simulink model "pv_array2"  (R2015a)
settings: Solver=ode45  StartTime=0.0  StopTime=10  RelTol=1e-3
undefined symbols (not defined in the file or in its folder): sigbuilder_block
libraries: powerlib x24
(part 1 of 2)
settings Model: Creator=Limon  LastModifiedBy=Limon

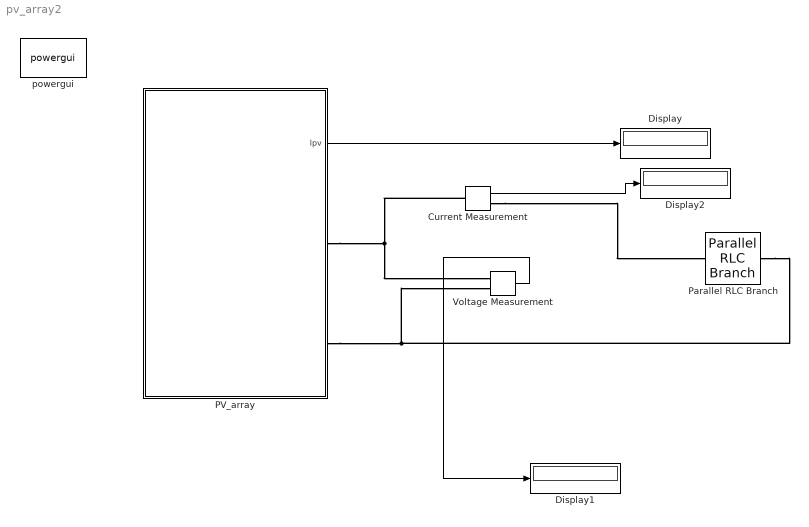
== system pv_array2 ==
  Current Measurement : powerlib/Measurements/Current Measurement  PhasorSimulation=off  OutputType=Complex  PSBequivalent=0
  Display : Display
  Display1 : Display
  Display2 : Display
  "PV_array " : Subsystem
  Parallel RLC Branch : powerlib/Elements/Parallel RLC Branch  LConnTagsString=a  RConnTagsString=__new0  BranchType=R  Resistance=1e3  Inductance=1e-3  SetiL0=off  InitialCurrent=0  Capacitance=1e-6  Setx0=off  InitialVoltage=0  Measurements=None
  Voltage Measurement : powerlib/Measurements/Voltage Measurement  PhasorSimulation=off  OutputType=Complex  PSBequivalent=0
  powergui : powerlib/powergui  Priority=1  SimulationMode=Discrete  SolverType=Tustin  SampleTime=.01  frequency=60  SPID=off  DisableSnubberDevices=off  DisableRonSwitches=off  DisableVfSwitches=off  SwTol=0  DisplayEquations=off  Interpol=off  methode=off  Ts=100  FunctionMessages=off  echomessages=off  HookPort=off  EnableUseOfTLC=off  x0status=blocks  frequencyindice=0  Pbase=100e6  ErrMax=0.0001  Iterations=50  UnitsV=kV  UnitsW=MW  buscounter=0  RestoreLinks=warning  ResistiveCurrentMeasurement=off  Frange=[0:2:500]  Ylog=off  Xlog=on  ShowGrid=off  save=off  variable=ZData  structure=MLFCDSTAT  ZoomFFT=off  StartTime=0.8  cycles=10  DisplayStyle=1  fundamental=50  FreqAxis=on  MaxFrequency=50000  frequencyindicesteady=1  RmsSteady=1  display=off
  wires:
  "PV_array "/1(Ipv) -> Display/1
  Voltage Measurement/1 -> Display1/1
  Current Measurement/1 -> Display2/1
  connections:
  "PV_array "/RConn1 -- Current Measurement/LConn1 -- Voltage Measurement/LConn1
  "PV_array "/RConn2 -- Parallel RLC Branch/RConn1 -- Voltage Measurement/LConn2
  Current Measurement/RConn1 -- Parallel RLC Branch/LConn1

== system pv_array2/PV_array  ==
  Irradiation : Subsystem
  PV module1 : Subsystem
  PV module10 : Subsystem
  PV module2 : Subsystem
  PV module3 : Subsystem
  PV module4 : Subsystem
  PV module5 : Subsystem
  PV module6 : Subsystem
  PV module7 : Subsystem
  PV module8 : Subsystem
  PV module9 : Subsystem
  + : PMIOPort  Port=1  Side=Right
  - : PMIOPort  Port=2  Side=Right
  Ipv : Outport
  wires:
  Irradiation/1(Irradiation) -> PV module1/1(Irradiation), PV module7/1(Irradiation), PV module10/1(Irradiation), PV module9/1(Irradiation), PV module5/1(Irradiation), PV module6/1(Irradiation), PV module8/1(Irradiation), PV module3/1(Irradiation), PV module4/1(Irradiation), PV module2/1(Irradiation)
  PV module9/1(Ipv) -> Ipv/1
  connections:
  PV module6/RConn1 -- PV module7/LConn1
  PV module9/RConn1 -- PV module10/LConn1
  PV module10/RConn1 -- PV module3/LConn1
  PV module5/RConn1 -- PV module6/LConn1
  PV module8/RConn1 -- -/RConn1
  PV module1/RConn1 -- PV module2/LConn1
  PV module9/LConn1 -- +/RConn1
  PV module4/LConn1 -- PV module2/RConn1
  PV module4/RConn1 -- PV module5/LConn1
  PV module1/LConn1 -- PV module3/RConn1
  PV module7/RConn1 -- PV module8/LConn1

== system pv_array2/PV_array /Irradiation ==
  Gain : Gain  Gain=1000
  Signal Builder : Subsystem  Tag=STV Subsys  LoadFcn=sigbuilder_block('load');  StartFcn=sigbuilder_block('start');  StopFcn=sigbuilder_block('stop');  ClipboardFcn=sigbuilder_block('clipboard');  mask(Sigbuilder block){}
      mask help: Simulink:masks:SigbuilderBlock_MD
      mask init:
      | if ~strcmp(get_param(bdroot(gcbh),'SimulationStatus'),'stopped') tuvar = sigbuilder_block('maskInit'); end
      settings: CopyFcn=sigbuilder_block('copy');  DeleteFcn=sigbuilder_block('delete');  ModelCloseFcn=sigbuilder_block('modelClose');  PreSaveFcn=sigbuilder_block('preSave');  PauseFcn=sigbuilder_block('pause');  ContinueFcn=sigbuilder_block('continue');  NameChangeFcn=sigbuilder_block('namechange');  OpenFcn=sigbuilder_block('open',[437.6 199.2 550.4 400 ]);  CloseFcn=sigbuilder_block('close');
      mask Display: plot(0, 0, 100, 100,[2, 2, 32, 32, 2], [68, 8, 8, 68, 68],[32, 2], [38, 38], [32, 19, 2],[53, 60, 44], [32, 17, 17, 2],[16, 16, 31, 31]);txt = getActiveGroup(gcbh);text(2, 100, txt,'verticalAlignment', 'top');
  Irradiation : Outport
  wires:
  Signal Builder/1(Signal 1) -> Gain/1
  Gain/1 -> Irradiation/1

== system pv_array2/PV_array /PV module1 ==
  Irradiation : Inport
  Display2 : Display
  PV module : Subsystem
  Temperature : Constant  Value=25
  VM1 : powerlib/Measurements/Voltage Measurement  PhasorSimulation=off  OutputType=Complex  PSBequivalent=0
  + : PMIOPort  Tag=PMCPort  Port=1  Side=Left
  - : PMIOPort  Tag=PMCPort  Port=2  Side=Right
  wires:
  Irradiation/1 -> PV module/2(Insol)
  Temperature/1 -> PV module/1(Temp)
  VM1/1 -> Display2/1
  connections:
  VM1/LConn1 -- +/RConn1 -- PV module/LConn1
  -/RConn1 -- VM1/LConn2 -- PV module/RConn1

== system pv_array2/PV_array /PV module10 ==
  Irradiation : Inport
  Display2 : Display
  PV module : Subsystem
  Temperature : Constant  Value=25
  VM1 : powerlib/Measurements/Voltage Measurement  PhasorSimulation=off  OutputType=Complex  PSBequivalent=0
  + : PMIOPort  Tag=PMCPort  Port=1  Side=Left
  - : PMIOPort  Tag=PMCPort  Port=2  Side=Right
  wires:
  Irradiation/1 -> PV module/2(Insol)
  Temperature/1 -> PV module/1(Temp)
  VM1/1 -> Display2/1
  connections:
  VM1/LConn1 -- +/RConn1 -- PV module/LConn1
  -/RConn1 -- VM1/LConn2 -- PV module/RConn1

== system pv_array2/PV_array /PV module2 ==
  Irradiation : Inport
  Display2 : Display
  PV module : Subsystem
  Temperature : Constant  Value=25
  VM1 : powerlib/Measurements/Voltage Measurement  PhasorSimulation=off  OutputType=Complex  PSBequivalent=0
  + : PMIOPort  Tag=PMCPort  Port=1  Side=Left
  - : PMIOPort  Tag=PMCPort  Port=2  Side=Right
  wires:
  Irradiation/1 -> PV module/2(Insol)
  Temperature/1 -> PV module/1(Temp)
  VM1/1 -> Display2/1
  connections:
  VM1/LConn1 -- +/RConn1 -- PV module/LConn1
  -/RConn1 -- VM1/LConn2 -- PV module/RConn1

== system pv_array2/PV_array /PV module3 ==
  Irradiation : Inport
  Display2 : Display
  PV module : Subsystem
  Temperature : Constant  Value=25
  VM1 : powerlib/Measurements/Voltage Measurement  PhasorSimulation=off  OutputType=Complex  PSBequivalent=0
  + : PMIOPort  Tag=PMCPort  Port=1  Side=Left
  - : PMIOPort  Tag=PMCPort  Port=2  Side=Right
  wires:
  Irradiation/1 -> PV module/2(Insol)
  Temperature/1 -> PV module/1(Temp)
  VM1/1 -> Display2/1
  connections:
  VM1/LConn1 -- +/RConn1 -- PV module/LConn1
  -/RConn1 -- VM1/LConn2 -- PV module/RConn1

== system pv_array2/PV_array /PV module4 ==
  Irradiation : Inport
  Display2 : Display
  PV module : Subsystem
  Temperature : Constant  Value=25
  VM1 : powerlib/Measurements/Voltage Measurement  PhasorSimulation=off  OutputType=Complex  PSBequivalent=0
  + : PMIOPort  Tag=PMCPort  Port=1  Side=Left
  - : PMIOPort  Tag=PMCPort  Port=2  Side=Right
  wires:
  Irradiation/1 -> PV module/2(Insol)
  Temperature/1 -> PV module/1(Temp)
  VM1/1 -> Display2/1
  connections:
  VM1/LConn1 -- +/RConn1 -- PV module/LConn1
  -/RConn1 -- VM1/LConn2 -- PV module/RConn1

== system pv_array2/PV_array /PV module5 ==
  Irradiation : Inport
  Display2 : Display
  PV module : Subsystem
  Temperature : Constant  Value=25
  VM1 : powerlib/Measurements/Voltage Measurement  PhasorSimulation=off  OutputType=Complex  PSBequivalent=0
  + : PMIOPort  Tag=PMCPort  Port=1  Side=Left
  - : PMIOPort  Tag=PMCPort  Port=2  Side=Right
  wires:
  Irradiation/1 -> PV module/2(Insol)
  Temperature/1 -> PV module/1(Temp)
  VM1/1 -> Display2/1
  connections:
  VM1/LConn1 -- +/RConn1 -- PV module/LConn1
  -/RConn1 -- VM1/LConn2 -- PV module/RConn1

== system pv_array2/PV_array /PV module6 ==
  Irradiation : Inport
  Display2 : Display
  PV module : Subsystem
  Temperature : Constant  Value=25
  VM1 : powerlib/Measurements/Voltage Measurement  PhasorSimulation=off  OutputType=Complex  PSBequivalent=0
  + : PMIOPort  Tag=PMCPort  Port=1  Side=Left
  - : PMIOPort  Tag=PMCPort  Port=2  Side=Right
  wires:
  Irradiation/1 -> PV module/2(Insol)
  Temperature/1 -> PV module/1(Temp)
  VM1/1 -> Display2/1
  connections:
  VM1/LConn1 -- +/RConn1 -- PV module/LConn1
  -/RConn1 -- VM1/LConn2 -- PV module/RConn1

== system pv_array2/PV_array /PV module7 ==
  Irradiation : Inport
  Display2 : Display
  PV module : Subsystem
  Temperature : Constant  Value=25
  VM1 : powerlib/Measurements/Voltage Measurement  PhasorSimulation=off  OutputType=Complex  PSBequivalent=0
  + : PMIOPort  Tag=PMCPort  Port=1  Side=Left
  - : PMIOPort  Tag=PMCPort  Port=2  Side=Right
  wires:
  Irradiation/1 -> PV module/2(Insol)
  Temperature/1 -> PV module/1(Temp)
  VM1/1 -> Display2/1
  connections:
  VM1/LConn1 -- +/RConn1 -- PV module/LConn1
  -/RConn1 -- VM1/LConn2 -- PV module/RConn1

== system pv_array2/PV_array /PV module8 ==
  Irradiation : Inport
  Display2 : Display
  PV module : Subsystem
  Temperature : Constant  Value=25
  VM1 : powerlib/Measurements/Voltage Measurement  PhasorSimulation=off  OutputType=Complex  PSBequivalent=0
  + : PMIOPort  Tag=PMCPort  Port=1  Side=Left
  - : PMIOPort  Tag=PMCPort  Port=2  Side=Right
  wires:
  Irradiation/1 -> PV module/2(Insol)
  Temperature/1 -> PV module/1(Temp)
  VM1/1 -> Display2/1
  connections:
  VM1/LConn1 -- +/RConn1 -- PV module/LConn1
  -/RConn1 -- VM1/LConn2 -- PV module/RConn1

== system pv_array2/PV_array /PV module9 ==
  Irradiation : Inport
  Display2 : Display
  PV module : Subsystem
  Temperature : Constant  Value=25
  VM1 : powerlib/Measurements/Voltage Measurement  PhasorSimulation=off  OutputType=Complex  PSBequivalent=0
  + : PMIOPort  Tag=PMCPort  Port=1  Side=Left
  - : PMIOPort  Tag=PMCPort  Port=2  Side=Right
  Ipv : Outport
  wires:
  Irradiation/1 -> PV module/2(Insol)
  Temperature/1 -> PV module/1(Temp)
  VM1/1 -> Display2/1
  PV module/1(Ipv) -> Ipv/1
  connections:
  VM1/LConn1 -- +/RConn1 -- PV module/LConn1
  -/RConn1 -- VM1/LConn2 -- PV module/RConn1

== system pv_array2/PV_array /Irradiation/Signal Builder ==
  Demux : Demux  Tag=STV Demux  Outputs=1
  FromWs : FromWorkspace  Tag=STV FromWs  VariableName=tuvar  SampleTime=0
      SigBuilderData=|
      | common.afterFinalStr = 'Extrapolate'
      | common.sampleTime = 0
      | dataSet.timeRange = [0 30]
      | dataSet.name = 'Group 1'
      | sbobj.Groups.Name = 'Group 1'
      | sbobj.Groups.Signals.Name = 'Signal 1'
      | sbobj.Groups.Signals.XData = [0 10 10 20 20 30]
      | sbobj.Groups.Signals.YData = [0.2 0.2 0.6 0.6 1 0.995]
      | sbobj.Groups.TimeRange = [0 30]
  Signal 1 : Outport  Tag=STV Outport
  wires:
  Demux/1 -> Signal 1/1
  FromWs/1 -> Demux/1

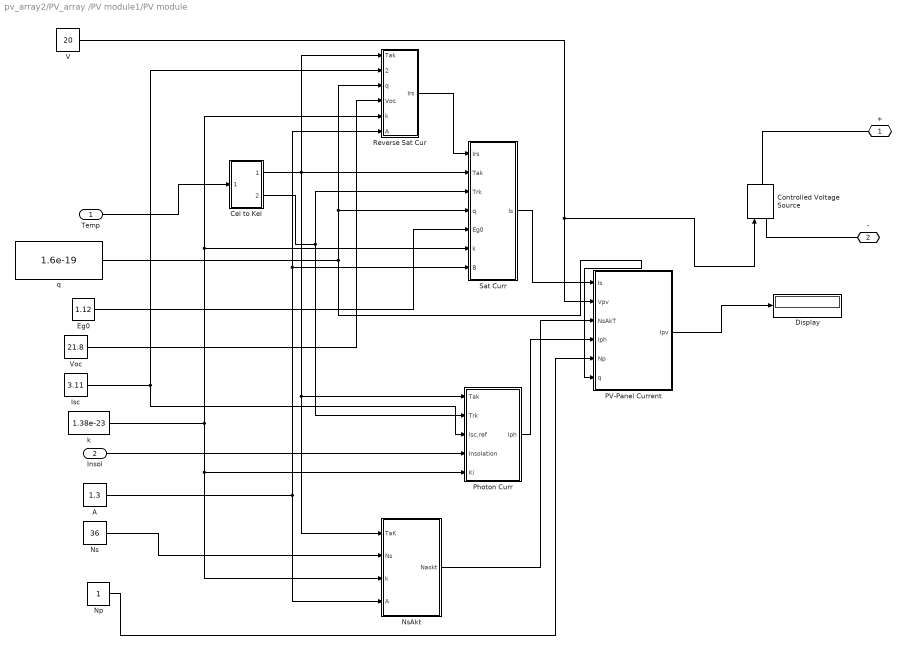
== system pv_array2/PV_array /PV module1/PV module ==
  Temp : Inport
  Insol : Inport  Port=2
  A : Constant  Value=1.3
  Cel to Kel : Subsystem
  Controlled Voltage Source : powerlib/Electrical Sources/Controlled Voltage Source  Initialize=on  Source_Type=AC  Amplitude=0  Phase=0  Frequency=0  Measurements=None
  Display : Display
  Eg0 : Constant  Value=1.12
  Isc : Constant  Value=3.11
  Np : Constant
  Ns : Constant  Value=36
  NsAkt : Subsystem
  PV-Panel Current : Subsystem
  "Photon Curr " : Subsystem
  "Reverse Sat Cur " : Subsystem
  Sat Curr : Subsystem
  V : Constant  Value=20
  Voc : Constant  Value=21.8
  k : Constant  Value=1.38e-23
  q : Constant  Value=1.6e-19
  + : PMIOPort  Port=1  Side=Left
  - : PMIOPort  Port=2  Side=Right
  wires:
  "Photon Curr "/1("Iph ") -> PV-Panel Current/4("Iph ")
  NsAkt/1(Naskt) -> PV-Panel Current/3(NsAkT)
  "Reverse Sat Cur "/1(Irs) -> Sat Curr/1(Irs)
  Cel to Kel/1("Tak ") -> "Photon Curr "/1("Tak "), NsAkt/1(TaK), "Reverse Sat Cur "/1("Tak "), Sat Curr/2(Tak)
  Sat Curr/1(Is) -> PV-Panel Current/1(Is)
  Temp/1 -> Cel to Kel/1("Top ")
  V/1 -> Controlled Voltage Source/1, PV-Panel Current/2("Vpv ")
  Ns/1 -> NsAkt/2(Ns)
  Cel to Kel/2("Trk ") -> "Photon Curr "/2(Trk), Sat Curr/3(Trk)
  Isc/1 -> "Reverse Sat Cur "/2("Isc ref "), "Photon Curr "/3(Isc,ref)
  q/1 -> Sat Curr/4(q), "Reverse Sat Cur "/3(q), PV-Panel Current/6(q)
  Voc/1 -> "Reverse Sat Cur "/4(Voc)
  k/1 -> Sat Curr/6(k), "Reverse Sat Cur "/5(k), NsAkt/3(k), "Photon Curr "/5(Ki)
  A/1 -> Sat Curr/7(B), "Reverse Sat Cur "/6("A "), NsAkt/4(A)
  Insol/1 -> "Photon Curr "/4("Insolation ")
  Np/1 -> PV-Panel Current/5(Np)
  Eg0/1 -> Sat Curr/5(Eg0)
  PV-Panel Current/1(Ipv) -> Display/1
  connections:
  +/RConn1 -- Controlled Voltage Source/RConn1
  -/RConn1 -- Controlled Voltage Source/LConn1

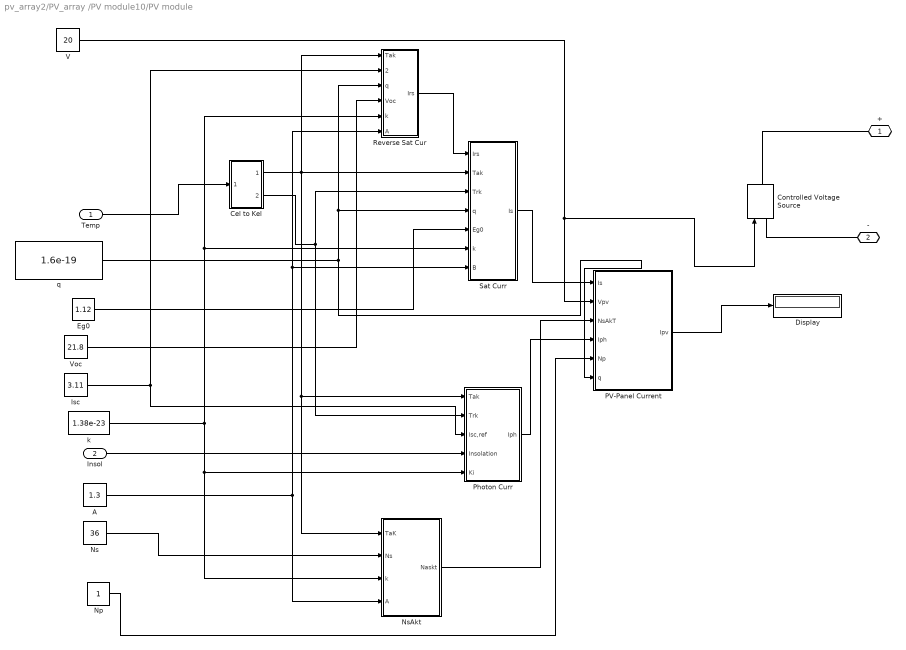
== system pv_array2/PV_array /PV module10/PV module ==
  Temp : Inport
  Insol : Inport  Port=2
  A : Constant  Value=1.3
  Cel to Kel : Subsystem
  Controlled Voltage Source : powerlib/Electrical Sources/Controlled Voltage Source  Initialize=on  Source_Type=AC  Amplitude=0  Phase=0  Frequency=0  Measurements=None
  Display : Display
  Eg0 : Constant  Value=1.12
  Isc : Constant  Value=3.11
  Np : Constant
  Ns : Constant  Value=36
  NsAkt : Subsystem
  PV-Panel Current : Subsystem
  "Photon Curr " : Subsystem
  "Reverse Sat Cur " : Subsystem
  Sat Curr : Subsystem
  V : Constant  Value=20
  Voc : Constant  Value=21.8
  k : Constant  Value=1.38e-23
  q : Constant  Value=1.6e-19
  + : PMIOPort  Port=1  Side=Left
  - : PMIOPort  Port=2  Side=Right
  wires:
  "Photon Curr "/1("Iph ") -> PV-Panel Current/4("Iph ")
  NsAkt/1(Naskt) -> PV-Panel Current/3(NsAkT)
  "Reverse Sat Cur "/1(Irs) -> Sat Curr/1(Irs)
  Cel to Kel/1("Tak ") -> "Photon Curr "/1("Tak "), NsAkt/1(TaK), "Reverse Sat Cur "/1("Tak "), Sat Curr/2(Tak)
  Sat Curr/1(Is) -> PV-Panel Current/1(Is)
  Temp/1 -> Cel to Kel/1("Top ")
  V/1 -> Controlled Voltage Source/1, PV-Panel Current/2("Vpv ")
  Ns/1 -> NsAkt/2(Ns)
  Cel to Kel/2("Trk ") -> "Photon Curr "/2(Trk), Sat Curr/3(Trk)
  Isc/1 -> "Reverse Sat Cur "/2("Isc ref "), "Photon Curr "/3(Isc,ref)
  q/1 -> Sat Curr/4(q), "Reverse Sat Cur "/3(q), PV-Panel Current/6(q)
  Voc/1 -> "Reverse Sat Cur "/4(Voc)
  k/1 -> Sat Curr/6(k), "Reverse Sat Cur "/5(k), NsAkt/3(k), "Photon Curr "/5(Ki)
  A/1 -> Sat Curr/7(B), "Reverse Sat Cur "/6("A "), NsAkt/4(A)
  Insol/1 -> "Photon Curr "/4("Insolation ")
  Np/1 -> PV-Panel Current/5(Np)
  Eg0/1 -> Sat Curr/5(Eg0)
  PV-Panel Current/1(Ipv) -> Display/1
  connections:
  +/RConn1 -- Controlled Voltage Source/RConn1
  -/RConn1 -- Controlled Voltage Source/LConn1

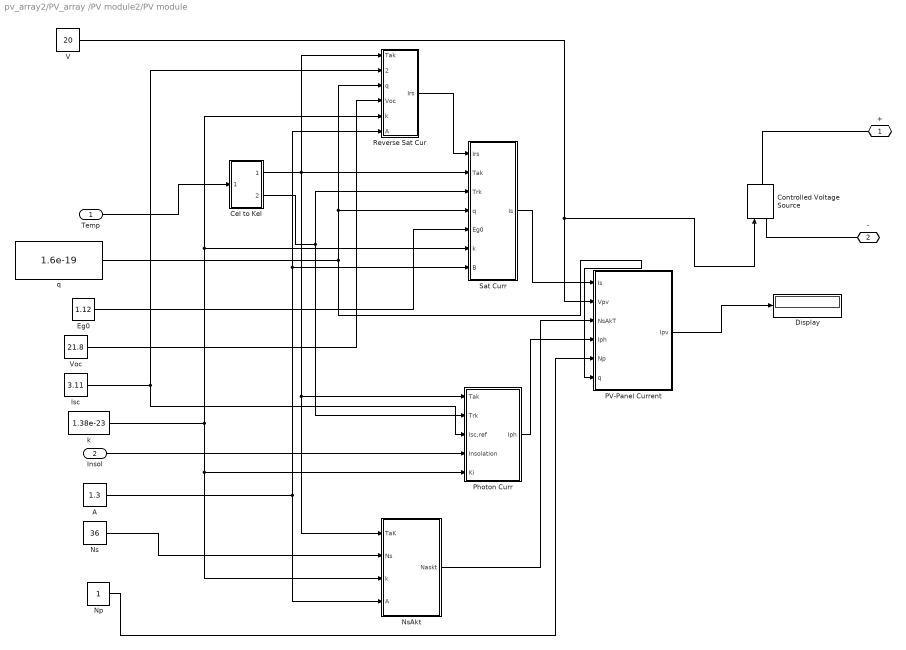
== system pv_array2/PV_array /PV module2/PV module ==
  Temp : Inport
  Insol : Inport  Port=2
  A : Constant  Value=1.3
  Cel to Kel : Subsystem
  Controlled Voltage Source : powerlib/Electrical Sources/Controlled Voltage Source  Initialize=on  Source_Type=AC  Amplitude=0  Phase=0  Frequency=0  Measurements=None
  Display : Display
  Eg0 : Constant  Value=1.12
  Isc : Constant  Value=3.11
  Np : Constant
  Ns : Constant  Value=36
  NsAkt : Subsystem
  PV-Panel Current : Subsystem
  "Photon Curr " : Subsystem
  "Reverse Sat Cur " : Subsystem
  Sat Curr : Subsystem
  V : Constant  Value=20
  Voc : Constant  Value=21.8
  k : Constant  Value=1.38e-23
  q : Constant  Value=1.6e-19
  + : PMIOPort  Port=1  Side=Left
  - : PMIOPort  Port=2  Side=Right
  wires:
  "Photon Curr "/1("Iph ") -> PV-Panel Current/4("Iph ")
  NsAkt/1(Naskt) -> PV-Panel Current/3(NsAkT)
  "Reverse Sat Cur "/1(Irs) -> Sat Curr/1(Irs)
  Cel to Kel/1("Tak ") -> "Photon Curr "/1("Tak "), NsAkt/1(TaK), "Reverse Sat Cur "/1("Tak "), Sat Curr/2(Tak)
  Sat Curr/1(Is) -> PV-Panel Current/1(Is)
  Temp/1 -> Cel to Kel/1("Top ")
  V/1 -> Controlled Voltage Source/1, PV-Panel Current/2("Vpv ")
  Ns/1 -> NsAkt/2(Ns)
  Cel to Kel/2("Trk ") -> "Photon Curr "/2(Trk), Sat Curr/3(Trk)
  Isc/1 -> "Reverse Sat Cur "/2("Isc ref "), "Photon Curr "/3(Isc,ref)
  q/1 -> Sat Curr/4(q), "Reverse Sat Cur "/3(q), PV-Panel Current/6(q)
  Voc/1 -> "Reverse Sat Cur "/4(Voc)
  k/1 -> Sat Curr/6(k), "Reverse Sat Cur "/5(k), NsAkt/3(k), "Photon Curr "/5(Ki)
  A/1 -> Sat Curr/7(B), "Reverse Sat Cur "/6("A "), NsAkt/4(A)
  Insol/1 -> "Photon Curr "/4("Insolation ")
  Np/1 -> PV-Panel Current/5(Np)
  Eg0/1 -> Sat Curr/5(Eg0)
  PV-Panel Current/1(Ipv) -> Display/1
  connections:
  +/RConn1 -- Controlled Voltage Source/RConn1
  -/RConn1 -- Controlled Voltage Source/LConn1

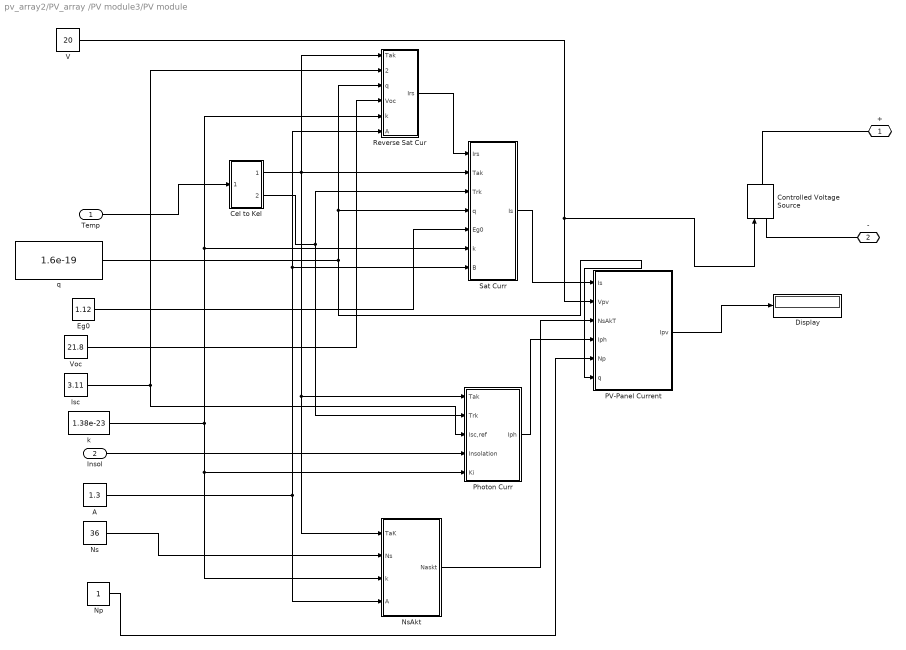
== system pv_array2/PV_array /PV module3/PV module ==
  Temp : Inport
  Insol : Inport  Port=2
  A : Constant  Value=1.3
  Cel to Kel : Subsystem
  Controlled Voltage Source : powerlib/Electrical Sources/Controlled Voltage Source  Initialize=on  Source_Type=AC  Amplitude=0  Phase=0  Frequency=0  Measurements=None
  Display : Display
  Eg0 : Constant  Value=1.12
  Isc : Constant  Value=3.11
  Np : Constant
  Ns : Constant  Value=36
  NsAkt : Subsystem
  PV-Panel Current : Subsystem
  "Photon Curr " : Subsystem
  "Reverse Sat Cur " : Subsystem
  Sat Curr : Subsystem
  V : Constant  Value=20
  Voc : Constant  Value=21.8
  k : Constant  Value=1.38e-23
  q : Constant  Value=1.6e-19
  + : PMIOPort  Port=1  Side=Left
  - : PMIOPort  Port=2  Side=Right
  wires:
  "Photon Curr "/1("Iph ") -> PV-Panel Current/4("Iph ")
  NsAkt/1(Naskt) -> PV-Panel Current/3(NsAkT)
  "Reverse Sat Cur "/1(Irs) -> Sat Curr/1(Irs)
  Cel to Kel/1("Tak ") -> "Photon Curr "/1("Tak "), NsAkt/1(TaK), "Reverse Sat Cur "/1("Tak "), Sat Curr/2(Tak)
  Sat Curr/1(Is) -> PV-Panel Current/1(Is)
  Temp/1 -> Cel to Kel/1("Top ")
  V/1 -> Controlled Voltage Source/1, PV-Panel Current/2("Vpv ")
  Ns/1 -> NsAkt/2(Ns)
  Cel to Kel/2("Trk ") -> "Photon Curr "/2(Trk), Sat Curr/3(Trk)
  Isc/1 -> "Reverse Sat Cur "/2("Isc ref "), "Photon Curr "/3(Isc,ref)
  q/1 -> Sat Curr/4(q), "Reverse Sat Cur "/3(q), PV-Panel Current/6(q)
  Voc/1 -> "Reverse Sat Cur "/4(Voc)
  k/1 -> Sat Curr/6(k), "Reverse Sat Cur "/5(k), NsAkt/3(k), "Photon Curr "/5(Ki)
  A/1 -> Sat Curr/7(B), "Reverse Sat Cur "/6("A "), NsAkt/4(A)
  Insol/1 -> "Photon Curr "/4("Insolation ")
  Np/1 -> PV-Panel Current/5(Np)
  Eg0/1 -> Sat Curr/5(Eg0)
  PV-Panel Current/1(Ipv) -> Display/1
  connections:
  +/RConn1 -- Controlled Voltage Source/RConn1
  -/RConn1 -- Controlled Voltage Source/LConn1

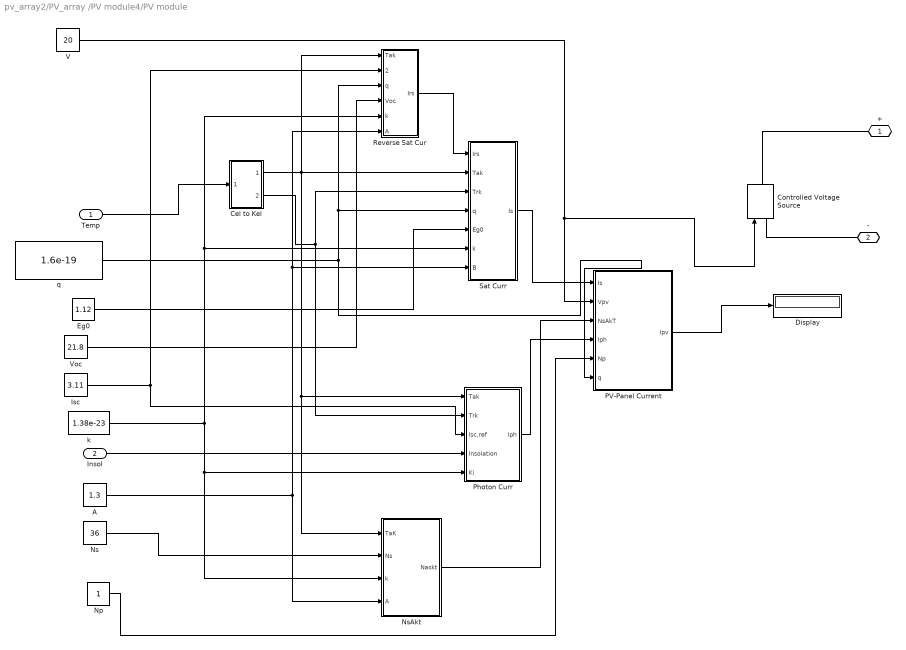
== system pv_array2/PV_array /PV module4/PV module ==
  Temp : Inport
  Insol : Inport  Port=2
  A : Constant  Value=1.3
  Cel to Kel : Subsystem
  Controlled Voltage Source : powerlib/Electrical Sources/Controlled Voltage Source  Initialize=on  Source_Type=AC  Amplitude=0  Phase=0  Frequency=0  Measurements=None
  Display : Display
  Eg0 : Constant  Value=1.12
  Isc : Constant  Value=3.11
  Np : Constant
  Ns : Constant  Value=36
  NsAkt : Subsystem
  PV-Panel Current : Subsystem
  "Photon Curr " : Subsystem
  "Reverse Sat Cur " : Subsystem
  Sat Curr : Subsystem
  V : Constant  Value=20
  Voc : Constant  Value=21.8
  k : Constant  Value=1.38e-23
  q : Constant  Value=1.6e-19
  + : PMIOPort  Port=1  Side=Left
  - : PMIOPort  Port=2  Side=Right
  wires:
  "Photon Curr "/1("Iph ") -> PV-Panel Current/4("Iph ")
  NsAkt/1(Naskt) -> PV-Panel Current/3(NsAkT)
  "Reverse Sat Cur "/1(Irs) -> Sat Curr/1(Irs)
  Cel to Kel/1("Tak ") -> "Photon Curr "/1("Tak "), NsAkt/1(TaK), "Reverse Sat Cur "/1("Tak "), Sat Curr/2(Tak)
  Sat Curr/1(Is) -> PV-Panel Current/1(Is)
  Temp/1 -> Cel to Kel/1("Top ")
  V/1 -> Controlled Voltage Source/1, PV-Panel Current/2("Vpv ")
  Ns/1 -> NsAkt/2(Ns)
  Cel to Kel/2("Trk ") -> "Photon Curr "/2(Trk), Sat Curr/3(Trk)
  Isc/1 -> "Reverse Sat Cur "/2("Isc ref "), "Photon Curr "/3(Isc,ref)
  q/1 -> Sat Curr/4(q), "Reverse Sat Cur "/3(q), PV-Panel Current/6(q)
  Voc/1 -> "Reverse Sat Cur "/4(Voc)
  k/1 -> Sat Curr/6(k), "Reverse Sat Cur "/5(k), NsAkt/3(k), "Photon Curr "/5(Ki)
  A/1 -> Sat Curr/7(B), "Reverse Sat Cur "/6("A "), NsAkt/4(A)
  Insol/1 -> "Photon Curr "/4("Insolation ")
  Np/1 -> PV-Panel Current/5(Np)
  Eg0/1 -> Sat Curr/5(Eg0)
  PV-Panel Current/1(Ipv) -> Display/1
  connections:
  +/RConn1 -- Controlled Voltage Source/RConn1
  -/RConn1 -- Controlled Voltage Source/LConn1

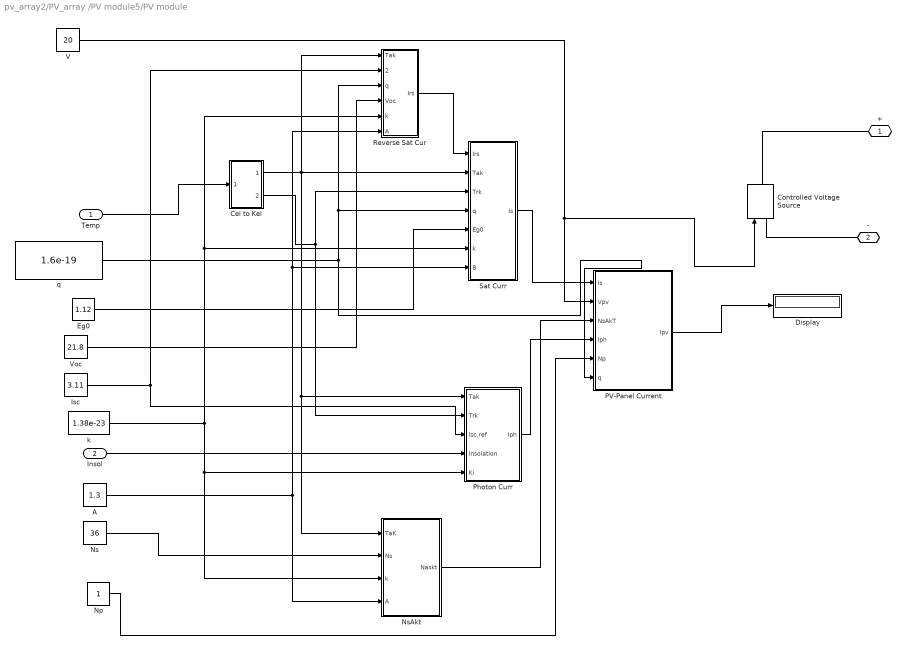
== system pv_array2/PV_array /PV module5/PV module ==
  Temp : Inport
  Insol : Inport  Port=2
  A : Constant  Value=1.3
  Cel to Kel : Subsystem
  Controlled Voltage Source : powerlib/Electrical Sources/Controlled Voltage Source  Initialize=on  Source_Type=AC  Amplitude=0  Phase=0  Frequency=0  Measurements=None
  Display : Display
  Eg0 : Constant  Value=1.12
  Isc : Constant  Value=3.11
  Np : Constant
  Ns : Constant  Value=36
  NsAkt : Subsystem
  PV-Panel Current : Subsystem
  "Photon Curr " : Subsystem
  "Reverse Sat Cur " : Subsystem
  Sat Curr : Subsystem
  V : Constant  Value=20
  Voc : Constant  Value=21.8
  k : Constant  Value=1.38e-23
  q : Constant  Value=1.6e-19
  + : PMIOPort  Port=1  Side=Left
  - : PMIOPort  Port=2  Side=Right
  wires:
  "Photon Curr "/1("Iph ") -> PV-Panel Current/4("Iph ")
  NsAkt/1(Naskt) -> PV-Panel Current/3(NsAkT)
  "Reverse Sat Cur "/1(Irs) -> Sat Curr/1(Irs)
  Cel to Kel/1("Tak ") -> "Photon Curr "/1("Tak "), NsAkt/1(TaK), "Reverse Sat Cur "/1("Tak "), Sat Curr/2(Tak)
  Sat Curr/1(Is) -> PV-Panel Current/1(Is)
  Temp/1 -> Cel to Kel/1("Top ")
  V/1 -> Controlled Voltage Source/1, PV-Panel Current/2("Vpv ")
  Ns/1 -> NsAkt/2(Ns)
  Cel to Kel/2("Trk ") -> "Photon Curr "/2(Trk), Sat Curr/3(Trk)
  Isc/1 -> "Reverse Sat Cur "/2("Isc ref "), "Photon Curr "/3(Isc,ref)
  q/1 -> Sat Curr/4(q), "Reverse Sat Cur "/3(q), PV-Panel Current/6(q)
  Voc/1 -> "Reverse Sat Cur "/4(Voc)
  k/1 -> Sat Curr/6(k), "Reverse Sat Cur "/5(k), NsAkt/3(k), "Photon Curr "/5(Ki)
  A/1 -> Sat Curr/7(B), "Reverse Sat Cur "/6("A "), NsAkt/4(A)
  Insol/1 -> "Photon Curr "/4("Insolation ")
  Np/1 -> PV-Panel Current/5(Np)
  Eg0/1 -> Sat Curr/5(Eg0)
  PV-Panel Current/1(Ipv) -> Display/1
  connections:
  +/RConn1 -- Controlled Voltage Source/RConn1
  -/RConn1 -- Controlled Voltage Source/LConn1

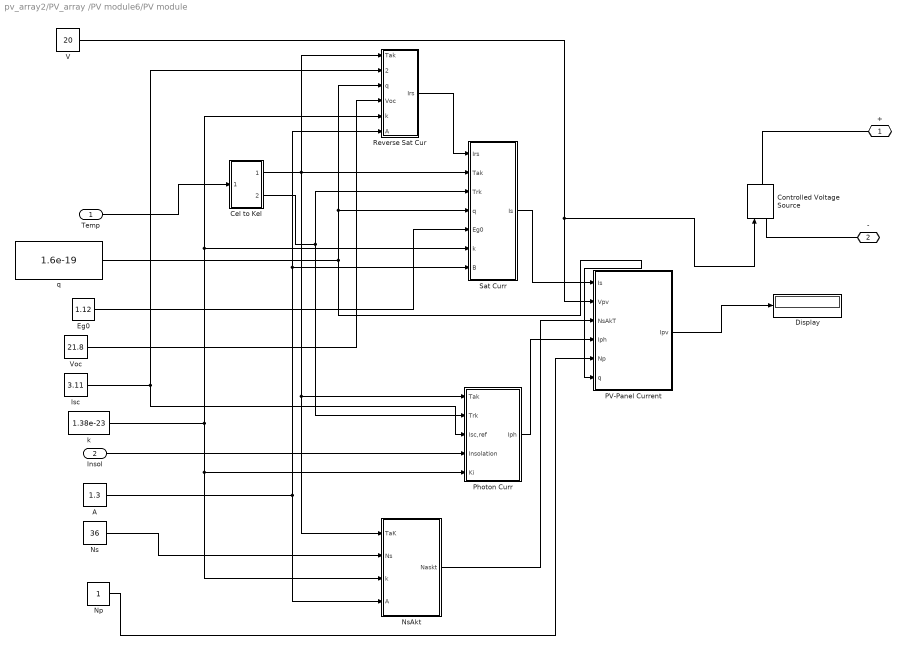
== system pv_array2/PV_array /PV module6/PV module ==
  Temp : Inport
  Insol : Inport  Port=2
  A : Constant  Value=1.3
  Cel to Kel : Subsystem
  Controlled Voltage Source : powerlib/Electrical Sources/Controlled Voltage Source  Initialize=on  Source_Type=AC  Amplitude=0  Phase=0  Frequency=0  Measurements=None
  Display : Display
  Eg0 : Constant  Value=1.12
  Isc : Constant  Value=3.11
  Np : Constant
  Ns : Constant  Value=36
  NsAkt : Subsystem
  PV-Panel Current : Subsystem
  "Photon Curr " : Subsystem
  "Reverse Sat Cur " : Subsystem
  Sat Curr : Subsystem
  V : Constant  Value=20
  Voc : Constant  Value=21.8
  k : Constant  Value=1.38e-23
  q : Constant  Value=1.6e-19
  + : PMIOPort  Port=1  Side=Left
  - : PMIOPort  Port=2  Side=Right
  wires:
  "Photon Curr "/1("Iph ") -> PV-Panel Current/4("Iph ")
  NsAkt/1(Naskt) -> PV-Panel Current/3(NsAkT)
  "Reverse Sat Cur "/1(Irs) -> Sat Curr/1(Irs)
  Cel to Kel/1("Tak ") -> "Photon Curr "/1("Tak "), NsAkt/1(TaK), "Reverse Sat Cur "/1("Tak "), Sat Curr/2(Tak)
  Sat Curr/1(Is) -> PV-Panel Current/1(Is)
  Temp/1 -> Cel to Kel/1("Top ")
  V/1 -> Controlled Voltage Source/1, PV-Panel Current/2("Vpv ")
  Ns/1 -> NsAkt/2(Ns)
  Cel to Kel/2("Trk ") -> "Photon Curr "/2(Trk), Sat Curr/3(Trk)
  Isc/1 -> "Reverse Sat Cur "/2("Isc ref "), "Photon Curr "/3(Isc,ref)
  q/1 -> Sat Curr/4(q), "Reverse Sat Cur "/3(q), PV-Panel Current/6(q)
  Voc/1 -> "Reverse Sat Cur "/4(Voc)
  k/1 -> Sat Curr/6(k), "Reverse Sat Cur "/5(k), NsAkt/3(k), "Photon Curr "/5(Ki)
  A/1 -> Sat Curr/7(B), "Reverse Sat Cur "/6("A "), NsAkt/4(A)
  Insol/1 -> "Photon Curr "/4("Insolation ")
  Np/1 -> PV-Panel Current/5(Np)
  Eg0/1 -> Sat Curr/5(Eg0)
  PV-Panel Current/1(Ipv) -> Display/1
  connections:
  +/RConn1 -- Controlled Voltage Source/RConn1
  -/RConn1 -- Controlled Voltage Source/LConn1

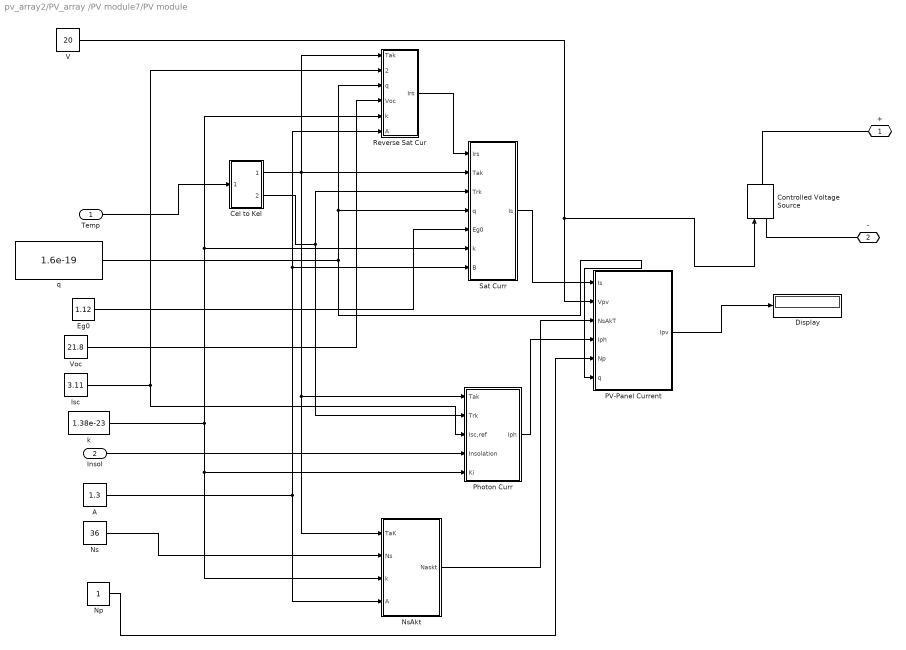
== system pv_array2/PV_array /PV module7/PV module ==
  Temp : Inport
  Insol : Inport  Port=2
  A : Constant  Value=1.3
  Cel to Kel : Subsystem
  Controlled Voltage Source : powerlib/Electrical Sources/Controlled Voltage Source  Initialize=on  Source_Type=AC  Amplitude=0  Phase=0  Frequency=0  Measurements=None
  Display : Display
  Eg0 : Constant  Value=1.12
  Isc : Constant  Value=3.11
  Np : Constant
  Ns : Constant  Value=36
  NsAkt : Subsystem
  PV-Panel Current : Subsystem
  "Photon Curr " : Subsystem
  "Reverse Sat Cur " : Subsystem
  Sat Curr : Subsystem
  V : Constant  Value=20
  Voc : Constant  Value=21.8
  k : Constant  Value=1.38e-23
  q : Constant  Value=1.6e-19
  + : PMIOPort  Port=1  Side=Left
  - : PMIOPort  Port=2  Side=Right
  wires:
  "Photon Curr "/1("Iph ") -> PV-Panel Current/4("Iph ")
  NsAkt/1(Naskt) -> PV-Panel Current/3(NsAkT)
  "Reverse Sat Cur "/1(Irs) -> Sat Curr/1(Irs)
  Cel to Kel/1("Tak ") -> "Photon Curr "/1("Tak "), NsAkt/1(TaK), "Reverse Sat Cur "/1("Tak "), Sat Curr/2(Tak)
  Sat Curr/1(Is) -> PV-Panel Current/1(Is)
  Temp/1 -> Cel to Kel/1("Top ")
  V/1 -> Controlled Voltage Source/1, PV-Panel Current/2("Vpv ")
  Ns/1 -> NsAkt/2(Ns)
  Cel to Kel/2("Trk ") -> "Photon Curr "/2(Trk), Sat Curr/3(Trk)
  Isc/1 -> "Reverse Sat Cur "/2("Isc ref "), "Photon Curr "/3(Isc,ref)
  q/1 -> Sat Curr/4(q), "Reverse Sat Cur "/3(q), PV-Panel Current/6(q)
  Voc/1 -> "Reverse Sat Cur "/4(Voc)
  k/1 -> Sat Curr/6(k), "Reverse Sat Cur "/5(k), NsAkt/3(k), "Photon Curr "/5(Ki)
  A/1 -> Sat Curr/7(B), "Reverse Sat Cur "/6("A "), NsAkt/4(A)
  Insol/1 -> "Photon Curr "/4("Insolation ")
  Np/1 -> PV-Panel Current/5(Np)
  Eg0/1 -> Sat Curr/5(Eg0)
  PV-Panel Current/1(Ipv) -> Display/1
  connections:
  +/RConn1 -- Controlled Voltage Source/RConn1
  -/RConn1 -- Controlled Voltage Source/LConn1

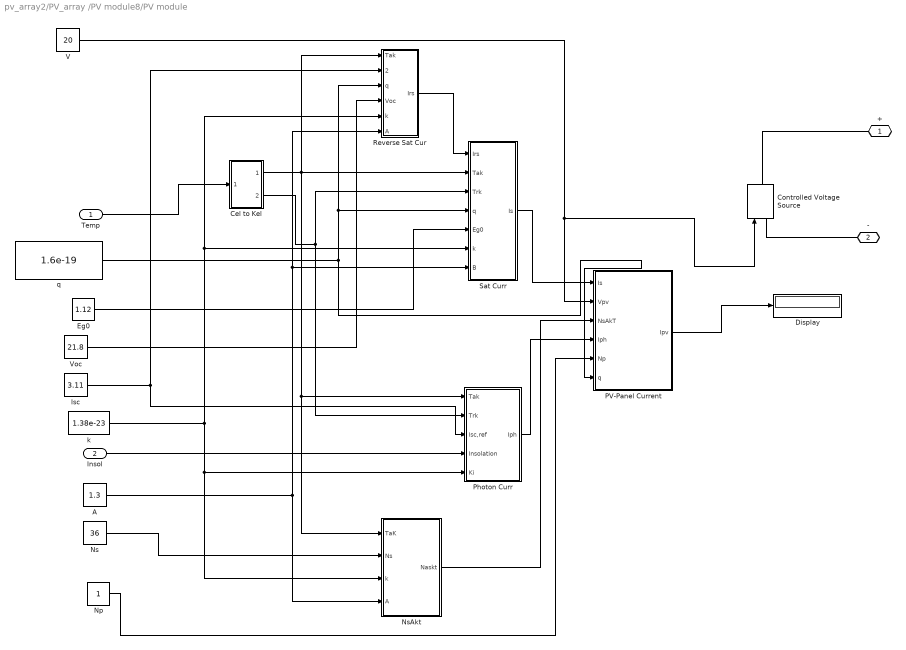
== system pv_array2/PV_array /PV module8/PV module ==
  Temp : Inport
  Insol : Inport  Port=2
  A : Constant  Value=1.3
  Cel to Kel : Subsystem
  Controlled Voltage Source : powerlib/Electrical Sources/Controlled Voltage Source  Initialize=on  Source_Type=AC  Amplitude=0  Phase=0  Frequency=0  Measurements=None
  Display : Display
  Eg0 : Constant  Value=1.12
  Isc : Constant  Value=3.11
  Np : Constant
  Ns : Constant  Value=36
  NsAkt : Subsystem
  PV-Panel Current : Subsystem
  "Photon Curr " : Subsystem
  "Reverse Sat Cur " : Subsystem
  Sat Curr : Subsystem
  V : Constant  Value=20
  Voc : Constant  Value=21.8
  k : Constant  Value=1.38e-23
  q : Constant  Value=1.6e-19
  + : PMIOPort  Port=1  Side=Left
  - : PMIOPort  Port=2  Side=Right
  wires:
  "Photon Curr "/1("Iph ") -> PV-Panel Current/4("Iph ")
  NsAkt/1(Naskt) -> PV-Panel Current/3(NsAkT)
  "Reverse Sat Cur "/1(Irs) -> Sat Curr/1(Irs)
  Cel to Kel/1("Tak ") -> "Photon Curr "/1("Tak "), NsAkt/1(TaK), "Reverse Sat Cur "/1("Tak "), Sat Curr/2(Tak)
  Sat Curr/1(Is) -> PV-Panel Current/1(Is)
  Temp/1 -> Cel to Kel/1("Top ")
  V/1 -> Controlled Voltage Source/1, PV-Panel Current/2("Vpv ")
  Ns/1 -> NsAkt/2(Ns)
  Cel to Kel/2("Trk ") -> "Photon Curr "/2(Trk), Sat Curr/3(Trk)
  Isc/1 -> "Reverse Sat Cur "/2("Isc ref "), "Photon Curr "/3(Isc,ref)
  q/1 -> Sat Curr/4(q), "Reverse Sat Cur "/3(q), PV-Panel Current/6(q)
  Voc/1 -> "Reverse Sat Cur "/4(Voc)
  k/1 -> Sat Curr/6(k), "Reverse Sat Cur "/5(k), NsAkt/3(k), "Photon Curr "/5(Ki)
  A/1 -> Sat Curr/7(B), "Reverse Sat Cur "/6("A "), NsAkt/4(A)
  Insol/1 -> "Photon Curr "/4("Insolation ")
  Np/1 -> PV-Panel Current/5(Np)
  Eg0/1 -> Sat Curr/5(Eg0)
  PV-Panel Current/1(Ipv) -> Display/1
  connections:
  +/RConn1 -- Controlled Voltage Source/RConn1
  -/RConn1 -- Controlled Voltage Source/LConn1

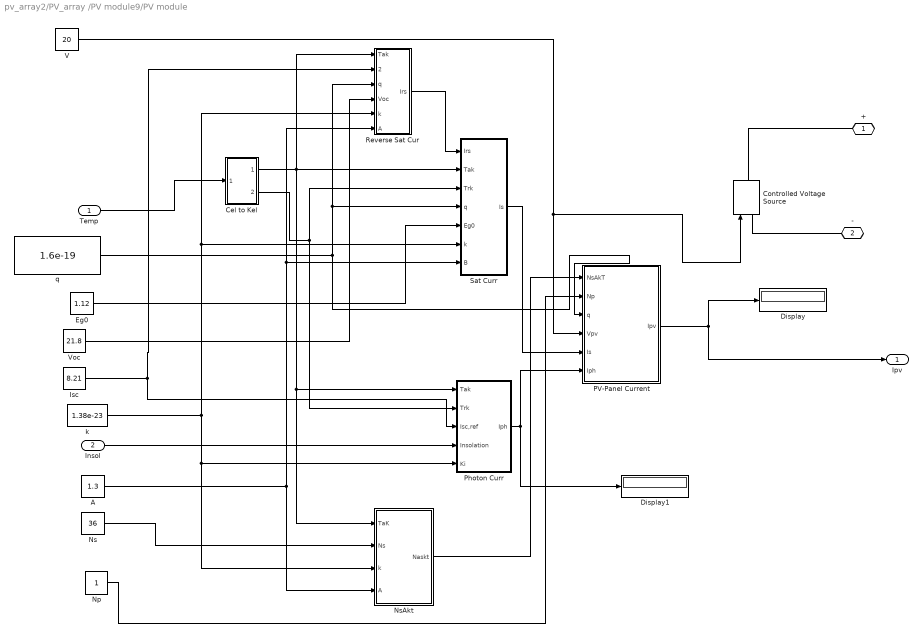
== system pv_array2/PV_array /PV module9/PV module ==
  Temp : Inport
  Insol : Inport  Port=2
  A : Constant  Value=1.3
  Cel to Kel : Subsystem
  Controlled Voltage Source : powerlib/Electrical Sources/Controlled Voltage Source  Initialize=on  Source_Type=AC  Amplitude=0  Phase=0  Frequency=0  Measurements=None
  Display : Display
  Display1 : Display
  Eg0 : Constant  Value=1.12
  Isc : Constant  Value=8.21
  Np : Constant
  Ns : Constant  Value=36
  NsAkt : Subsystem
  PV-Panel Current : Subsystem
  "Photon Curr " : Subsystem
  "Reverse Sat Cur " : Subsystem
  Sat Curr : Subsystem
  V : Constant  Value=20
  Voc : Constant  Value=21.8
  k : Constant  Value=1.38e-23
  q : Constant  Value=1.6e-19
  + : PMIOPort  Port=1  Side=Left
  - : PMIOPort  Port=2  Side=Right
  Ipv : Outport
  wires:
  NsAkt/1(Naskt) -> PV-Panel Current/1(NsAkT)
  "Reverse Sat Cur "/1(Irs) -> Sat Curr/1(Irs)
  Cel to Kel/1("Tak ") -> "Photon Curr "/1("Tak "), NsAkt/1(TaK), "Reverse Sat Cur "/1("Tak "), Sat Curr/2(Tak)
  Sat Curr/1(Is) -> PV-Panel Current/5(Is)
  Temp/1 -> Cel to Kel/1("Top ")
  V/1 -> Controlled Voltage Source/1, PV-Panel Current/4("Vpv ")
  Ns/1 -> NsAkt/2(Ns)
  Cel to Kel/2("Trk ") -> "Photon Curr "/2(Trk), Sat Curr/3(Trk)
  Isc/1 -> "Reverse Sat Cur "/2("Isc ref "), "Photon Curr "/3(Isc,ref)
  q/1 -> Sat Curr/4(q), "Reverse Sat Cur "/3(q), PV-Panel Current/3(q)
  Voc/1 -> "Reverse Sat Cur "/4(Voc)
  k/1 -> Sat Curr/6(k), "Reverse Sat Cur "/5(k), NsAkt/3(k), "Photon Curr "/5(Ki)
  A/1 -> Sat Curr/7(B), "Reverse Sat Cur "/6("A "), NsAkt/4(A)
  Insol/1 -> "Photon Curr "/4("Insolation ")
  Np/1 -> PV-Panel Current/2(Np)
  Eg0/1 -> Sat Curr/5(Eg0)
  PV-Panel Current/1(Ipv) -> Display/1, Ipv/1
  "Photon Curr "/1("Iph ") -> PV-Panel Current/6("Iph "), Display1/1
  connections:
  +/RConn1 -- Controlled Voltage Source/RConn1
  -/RConn1 -- Controlled Voltage Source/LConn1

== system pv_array2/PV_array /PV module1/PV module/Cel to Kel ==
  "Top " : Inport
  Add : Sum
  Add1 : Sum
  Cel to Kel : Constant  Value=273
  T(ref ^C)1 : Constant  Value=25
  "Tak " : Outport
  "Trk " : Outport  Port=2
  wires:
  Add/1 -> "Tak "/1
  Add1/1 -> "Trk "/1
  T(ref ^C)1/1 -> Add1/1
  Cel to Kel/1 -> Add1/2, Add/2
  "Top "/1 -> Add/1

== system pv_array2/PV_array /PV module1/PV module/NsAkt ==
  TaK : Inport
  Ns : Inport  Port=2
  k : Inport  Port=3
  A : Inport  Port=4
  Product : Product  Inputs=4
  Naskt : Outport
  wires:
  Product/1 -> Naskt/1
  TaK/1 -> Product/4
  Ns/1 -> Product/1
  k/1 -> Product/2
  A/1 -> Product/3

== system pv_array2/PV_array /PV module1/PV module/PV-Panel Current ==
  Is : Inport
  "Vpv " : Inport  Port=2
  NsAkT : Inport  Port=3
  "Iph " : Inport  Port=4
  Np : Inport  Port=5
  q : Inport  Port=6
  Fcn : Fcn  Expr=u(7)*u(2)-u(6)*u(2)*(exp((u(3)*(u(4)+u(5))/u(1)))-1)
  Mux : Mux  Inputs=7
  Rs : Gain  Gain=0.45
  Ipv : Outport
  wires:
  NsAkT/1 -> Mux/1
  Fcn/1 -> Ipv/1, Rs/1
  Rs/1 -> Mux/5
  "Iph "/1 -> Mux/7
  Is/1 -> Mux/6
  "Vpv "/1 -> Mux/4
  Mux/1 -> Fcn/1
  Np/1 -> Mux/2
  q/1 -> Mux/3

== system pv_array2/PV_array /PV module1/PV module/Photon Curr  ==
  "Tak " : Inport
  Trk : Inport  Port=2
  Isc,ref : Inport  Port=3
  "Insolation " : Inport  Port=4
  Ki : Inport  Port=5
  " " : Constant  Value=1000
  Divide : Product  Inputs=*/
  Product : Product
  Product1 : Product
  Sum1 : Sum  Inputs=|++
  Sum2 : Sum  Inputs=|+-
  "Iph " : Outport
  wires:
  "Tak "/1 -> Sum2/1
  Trk/1 -> Sum2/2
  Sum2/1 -> Product/2
  Product/1 -> Sum1/1
  Isc,ref/1 -> Sum1/2
  "Insolation "/1 -> Divide/1
  " "/1 -> Divide/2
  Divide/1 -> Product1/1
  Product1/1 -> "Iph "/1
  Sum1/1 -> Product1/2
  Ki/1 -> Product/1

== system pv_array2/PV_array /PV module1/PV module/Reverse Sat Cur  ==
  "Tak " : Inport
  "Isc ref " : Inport  Port=2
  q : Inport  Port=3
  Voc : Inport  Port=4
  k : Inport  Port=5
  "A " : Inport  Port=6
  "Constant " : Constant
  Divide : Product  Inputs=**////
  Fcn : Fcn  Expr=u(1)/(exp(u(2))-u(3))
  Mux : Mux  Inputs=3
  "Ns " : Constant  Value=36
  Irs : Outport
  wires:
  "Tak "/1 -> Divide/6
  "Ns "/1 -> Divide/4
  "Isc ref "/1 -> Mux/1
  Divide/1 -> Mux/2
  "Constant "/1 -> Mux/3
  Mux/1 -> Fcn/1
  Fcn/1 -> Irs/1
  q/1 -> Divide/1
  Voc/1 -> Divide/2
  k/1 -> Divide/3
  "A "/1 -> Divide/5

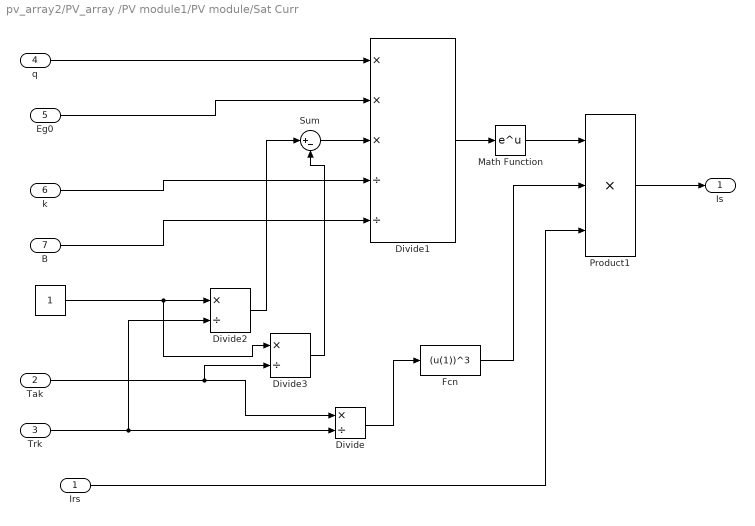
== system pv_array2/PV_array /PV module1/PV module/Sat Curr ==
  Irs : Inport
  Tak : Inport  Port=2
  Trk : Inport  Port=3
  q : Inport  Port=4
  Eg0 : Inport  Port=5
  k : Inport  Port=6
  B : Inport  Port=7
  " " : Constant
  Divide : Product  Inputs=*/
  Divide1 : Product  Inputs=***//
  Divide2 : Product  Inputs=*/
  Divide3 : Product  Inputs=*/
  Fcn : Fcn  Expr=(u(1))^3
  Math Function : Math  SaturateOnIntegerOverflow=on
  Product1 : Product  Inputs=3
  Sum : Sum  Inputs=|+-
  Is : Outport
  wires:
  Sum/1 -> Divide1/3
  Fcn/1 -> Product1/2
  Divide/1 -> Fcn/1
  Product1/1 -> Is/1
  Math Function/1 -> Product1/1
  Divide1/1 -> Math Function/1
  Tak/1 -> Divide3/2, Divide/1
  Irs/1 -> Product1/3
  " "/1 -> Divide3/1, Divide2/1
  Trk/1 -> Divide2/2, Divide/2
  Divide2/1 -> Sum/1
  Divide3/1 -> Sum/2
  q/1 -> Divide1/1
  Eg0/1 -> Divide1/2
  k/1 -> Divide1/4
  B/1 -> Divide1/5

== system pv_array2/PV_array /PV module10/PV module/Cel to Kel ==
  "Top " : Inport
  Add : Sum
  Add1 : Sum
  Cel to Kel : Constant  Value=273
  T(ref ^C)1 : Constant  Value=25
  "Tak " : Outport
  "Trk " : Outport  Port=2
  wires:
  Add/1 -> "Tak "/1
  Add1/1 -> "Trk "/1
  T(ref ^C)1/1 -> Add1/1
  Cel to Kel/1 -> Add1/2, Add/2
  "Top "/1 -> Add/1

== system pv_array2/PV_array /PV module10/PV module/NsAkt ==
  TaK : Inport
  Ns : Inport  Port=2
  k : Inport  Port=3
  A : Inport  Port=4
  Product : Product  Inputs=4
  Naskt : Outport
  wires:
  Product/1 -> Naskt/1
  TaK/1 -> Product/4
  Ns/1 -> Product/1
  k/1 -> Product/2
  A/1 -> Product/3

== system pv_array2/PV_array /PV module10/PV module/PV-Panel Current ==
  Is : Inport
  "Vpv " : Inport  Port=2
  NsAkT : Inport  Port=3
  "Iph " : Inport  Port=4
  Np : Inport  Port=5
  q : Inport  Port=6
  Fcn : Fcn  Expr=u(7)*u(2)-u(6)*u(2)*(exp((u(3)*(u(4)+u(5))/u(1)))-1)
  Mux : Mux  Inputs=7
  Rs : Gain  Gain=0.45
  Ipv : Outport
  wires:
  NsAkT/1 -> Mux/1
  Fcn/1 -> Ipv/1, Rs/1
  Rs/1 -> Mux/5
  "Iph "/1 -> Mux/7
  Is/1 -> Mux/6
  "Vpv "/1 -> Mux/4
  Mux/1 -> Fcn/1
  Np/1 -> Mux/2
  q/1 -> Mux/3

== system pv_array2/PV_array /PV module10/PV module/Photon Curr  ==
  "Tak " : Inport
  Trk : Inport  Port=2
  Isc,ref : Inport  Port=3
  "Insolation " : Inport  Port=4
  Ki : Inport  Port=5
  " " : Constant  Value=1000
  Divide : Product  Inputs=*/
  Product : Product
  Product1 : Product
  Sum1 : Sum  Inputs=|++
  Sum2 : Sum  Inputs=|+-
  "Iph " : Outport
  wires:
  "Tak "/1 -> Sum2/1
  Trk/1 -> Sum2/2
  Sum2/1 -> Product/2
  Product/1 -> Sum1/1
  Isc,ref/1 -> Sum1/2
  "Insolation "/1 -> Divide/1
  " "/1 -> Divide/2
  Divide/1 -> Product1/1
  Product1/1 -> "Iph "/1
  Sum1/1 -> Product1/2
  Ki/1 -> Product/1

== system pv_array2/PV_array /PV module10/PV module/Reverse Sat Cur  ==
  "Tak " : Inport
  "Isc ref " : Inport  Port=2
  q : Inport  Port=3
  Voc : Inport  Port=4
  k : Inport  Port=5
  "A " : Inport  Port=6
  "Constant " : Constant
  Divide : Product  Inputs=**////
  Fcn : Fcn  Expr=u(1)/(exp(u(2))-u(3))
  Mux : Mux  Inputs=3
  "Ns " : Constant  Value=36
  Irs : Outport
  wires:
  "Tak "/1 -> Divide/6
  "Ns "/1 -> Divide/4
  "Isc ref "/1 -> Mux/1
  Divide/1 -> Mux/2
  "Constant "/1 -> Mux/3
  Mux/1 -> Fcn/1
  Fcn/1 -> Irs/1
  q/1 -> Divide/1
  Voc/1 -> Divide/2
  k/1 -> Divide/3
  "A "/1 -> Divide/5

== system pv_array2/PV_array /PV module10/PV module/Sat Curr ==
  Irs : Inport
  Tak : Inport  Port=2
  Trk : Inport  Port=3
  q : Inport  Port=4
  Eg0 : Inport  Port=5
  k : Inport  Port=6
  B : Inport  Port=7
  " " : Constant
  Divide : Product  Inputs=*/
  Divide1 : Product  Inputs=***//
  Divide2 : Product  Inputs=*/
  Divide3 : Product  Inputs=*/
  Fcn : Fcn  Expr=(u(1))^3
  Math Function : Math  SaturateOnIntegerOverflow=on
  Product1 : Product  Inputs=3
  Sum : Sum  Inputs=|+-
  Is : Outport
  wires:
  Sum/1 -> Divide1/3
  Fcn/1 -> Product1/2
  Divide/1 -> Fcn/1
  Product1/1 -> Is/1
  Math Function/1 -> Product1/1
  Divide1/1 -> Math Function/1
  Tak/1 -> Divide3/2, Divide/1
  Irs/1 -> Product1/3
  " "/1 -> Divide3/1, Divide2/1
  Trk/1 -> Divide2/2, Divide/2
  Divide2/1 -> Sum/1
  Divide3/1 -> Sum/2
  q/1 -> Divide1/1
  Eg0/1 -> Divide1/2
  k/1 -> Divide1/4
  B/1 -> Divide1/5

== system pv_array2/PV_array /PV module2/PV module/Cel to Kel ==
  "Top " : Inport
  Add : Sum
  Add1 : Sum
  Cel to Kel : Constant  Value=273
  T(ref ^C)1 : Constant  Value=25
  "Tak " : Outport
  "Trk " : Outport  Port=2
  wires:
  Add/1 -> "Tak "/1
  Add1/1 -> "Trk "/1
  T(ref ^C)1/1 -> Add1/1
  Cel to Kel/1 -> Add1/2, Add/2
  "Top "/1 -> Add/1

== system pv_array2/PV_array /PV module2/PV module/NsAkt ==
  TaK : Inport
  Ns : Inport  Port=2
  k : Inport  Port=3
  A : Inport  Port=4
  Product : Product  Inputs=4
  Naskt : Outport
  wires:
  Product/1 -> Naskt/1
  TaK/1 -> Product/4
  Ns/1 -> Product/1
  k/1 -> Product/2
  A/1 -> Product/3

== system pv_array2/PV_array /PV module2/PV module/PV-Panel Current ==
  Is : Inport
  "Vpv " : Inport  Port=2
  NsAkT : Inport  Port=3
  "Iph " : Inport  Port=4
  Np : Inport  Port=5
  q : Inport  Port=6
  Fcn : Fcn  Expr=u(7)*u(2)-u(6)*u(2)*(exp((u(3)*(u(4)+u(5))/u(1)))-1)
  Mux : Mux  Inputs=7
  Rs : Gain  Gain=0.45
  Ipv : Outport
  wires:
  NsAkT/1 -> Mux/1
  Fcn/1 -> Ipv/1, Rs/1
  Rs/1 -> Mux/5
  "Iph "/1 -> Mux/7
  Is/1 -> Mux/6
  "Vpv "/1 -> Mux/4
  Mux/1 -> Fcn/1
  Np/1 -> Mux/2
  q/1 -> Mux/3

== system pv_array2/PV_array /PV module2/PV module/Photon Curr  ==
  "Tak " : Inport
  Trk : Inport  Port=2
  Isc,ref : Inport  Port=3
  "Insolation " : Inport  Port=4
  Ki : Inport  Port=5
  " " : Constant  Value=1000
  Divide : Product  Inputs=*/
  Product : Product
  Product1 : Product
  Sum1 : Sum  Inputs=|++
  Sum2 : Sum  Inputs=|+-
  "Iph " : Outport
  wires:
  "Tak "/1 -> Sum2/1
  Trk/1 -> Sum2/2
  Sum2/1 -> Product/2
  Product/1 -> Sum1/1
  Isc,ref/1 -> Sum1/2
  "Insolation "/1 -> Divide/1
  " "/1 -> Divide/2
  Divide/1 -> Product1/1
  Product1/1 -> "Iph "/1
  Sum1/1 -> Product1/2
  Ki/1 -> Product/1

== system pv_array2/PV_array /PV module2/PV module/Reverse Sat Cur  ==
  "Tak " : Inport
  "Isc ref " : Inport  Port=2
  q : Inport  Port=3
  Voc : Inport  Port=4
  k : Inport  Port=5
  "A " : Inport  Port=6
  "Constant " : Constant
  Divide : Product  Inputs=**////
  Fcn : Fcn  Expr=u(1)/(exp(u(2))-u(3))
  Mux : Mux  Inputs=3
  "Ns " : Constant  Value=36
  Irs : Outport
  wires:
  "Tak "/1 -> Divide/6
  "Ns "/1 -> Divide/4
  "Isc ref "/1 -> Mux/1
  Divide/1 -> Mux/2
  "Constant "/1 -> Mux/3
  Mux/1 -> Fcn/1
  Fcn/1 -> Irs/1
  q/1 -> Divide/1
  Voc/1 -> Divide/2
  k/1 -> Divide/3
  "A "/1 -> Divide/5

== system pv_array2/PV_array /PV module2/PV module/Sat Curr ==
  Irs : Inport
  Tak : Inport  Port=2
  Trk : Inport  Port=3
  q : Inport  Port=4
  Eg0 : Inport  Port=5
  k : Inport  Port=6
  B : Inport  Port=7
  " " : Constant
  Divide : Product  Inputs=*/
  Divide1 : Product  Inputs=***//
  Divide2 : Product  Inputs=*/
  Divide3 : Product  Inputs=*/
  Fcn : Fcn  Expr=(u(1))^3
  Math Function : Math  SaturateOnIntegerOverflow=on
  Product1 : Product  Inputs=3
  Sum : Sum  Inputs=|+-
  Is : Outport
  wires:
  Sum/1 -> Divide1/3
  Fcn/1 -> Product1/2
  Divide/1 -> Fcn/1
  Product1/1 -> Is/1
  Math Function/1 -> Product1/1
  Divide1/1 -> Math Function/1
  Tak/1 -> Divide3/2, Divide/1
  Irs/1 -> Product1/3
  " "/1 -> Divide3/1, Divide2/1
  Trk/1 -> Divide2/2, Divide/2
  Divide2/1 -> Sum/1
  Divide3/1 -> Sum/2
  q/1 -> Divide1/1
  Eg0/1 -> Divide1/2
  k/1 -> Divide1/4
  B/1 -> Divide1/5

== system pv_array2/PV_array /PV module3/PV module/Cel to Kel ==
  "Top " : Inport
  Add : Sum
  Add1 : Sum
  Cel to Kel : Constant  Value=273
  T(ref ^C)1 : Constant  Value=25
  "Tak " : Outport
  "Trk " : Outport  Port=2
  wires:
  Add/1 -> "Tak "/1
  Add1/1 -> "Trk "/1
  T(ref ^C)1/1 -> Add1/1
  Cel to Kel/1 -> Add1/2, Add/2
  "Top "/1 -> Add/1

== system pv_array2/PV_array /PV module3/PV module/NsAkt ==
  TaK : Inport
  Ns : Inport  Port=2
  k : Inport  Port=3
  A : Inport  Port=4
  Product : Product  Inputs=4
  Naskt : Outport
  wires:
  Product/1 -> Naskt/1
  TaK/1 -> Product/4
  Ns/1 -> Product/1
  k/1 -> Product/2
  A/1 -> Product/3

== system pv_array2/PV_array /PV module3/PV module/PV-Panel Current ==
  Is : Inport
  "Vpv " : Inport  Port=2
  NsAkT : Inport  Port=3
  "Iph " : Inport  Port=4
  Np : Inport  Port=5
  q : Inport  Port=6
  Fcn : Fcn  Expr=u(7)*u(2)-u(6)*u(2)*(exp((u(3)*(u(4)+u(5))/u(1)))-1)
  Mux : Mux  Inputs=7
  Rs : Gain  Gain=0.45
  Ipv : Outport
  wires:
  NsAkT/1 -> Mux/1
  Fcn/1 -> Ipv/1, Rs/1
  Rs/1 -> Mux/5
  "Iph "/1 -> Mux/7
  Is/1 -> Mux/6
  "Vpv "/1 -> Mux/4
  Mux/1 -> Fcn/1
  Np/1 -> Mux/2
  q/1 -> Mux/3

== system pv_array2/PV_array /PV module3/PV module/Photon Curr  ==
  "Tak " : Inport
  Trk : Inport  Port=2
  Isc,ref : Inport  Port=3
  "Insolation " : Inport  Port=4
  Ki : Inport  Port=5
  " " : Constant  Value=1000
  Divide : Product  Inputs=*/
  Product : Product
  Product1 : Product
  Sum1 : Sum  Inputs=|++
  Sum2 : Sum  Inputs=|+-
  "Iph " : Outport
  wires:
  "Tak "/1 -> Sum2/1
  Trk/1 -> Sum2/2
  Sum2/1 -> Product/2
  Product/1 -> Sum1/1
  Isc,ref/1 -> Sum1/2
  "Insolation "/1 -> Divide/1
  " "/1 -> Divide/2
  Divide/1 -> Product1/1
  Product1/1 -> "Iph "/1
  Sum1/1 -> Product1/2
  Ki/1 -> Product/1

== system pv_array2/PV_array /PV module3/PV module/Reverse Sat Cur  ==
  "Tak " : Inport
  "Isc ref " : Inport  Port=2
  q : Inport  Port=3
  Voc : Inport  Port=4
  k : Inport  Port=5
  "A " : Inport  Port=6
  "Constant " : Constant
  Divide : Product  Inputs=**////
  Fcn : Fcn  Expr=u(1)/(exp(u(2))-u(3))
  Mux : Mux  Inputs=3
  "Ns " : Constant  Value=36
  Irs : Outport
  wires:
  "Tak "/1 -> Divide/6
  "Ns "/1 -> Divide/4
  "Isc ref "/1 -> Mux/1
  Divide/1 -> Mux/2
  "Constant "/1 -> Mux/3
  Mux/1 -> Fcn/1
  Fcn/1 -> Irs/1
  q/1 -> Divide/1
  Voc/1 -> Divide/2
  k/1 -> Divide/3
  "A "/1 -> Divide/5

== system pv_array2/PV_array /PV module3/PV module/Sat Curr ==
  Irs : Inport
  Tak : Inport  Port=2
  Trk : Inport  Port=3
  q : Inport  Port=4
  Eg0 : Inport  Port=5
  k : Inport  Port=6
  B : Inport  Port=7
  " " : Constant
  Divide : Product  Inputs=*/
  Divide1 : Product  Inputs=***//
  Divide2 : Product  Inputs=*/
  Divide3 : Product  Inputs=*/
  Fcn : Fcn  Expr=(u(1))^3
  Math Function : Math  SaturateOnIntegerOverflow=on
  Product1 : Product  Inputs=3
  Sum : Sum  Inputs=|+-
  Is : Outport
  wires:
  Sum/1 -> Divide1/3
  Fcn/1 -> Product1/2
  Divide/1 -> Fcn/1
  Product1/1 -> Is/1
  Math Function/1 -> Product1/1
  Divide1/1 -> Math Function/1
  Tak/1 -> Divide3/2, Divide/1
  Irs/1 -> Product1/3
  " "/1 -> Divide3/1, Divide2/1
  Trk/1 -> Divide2/2, Divide/2
  Divide2/1 -> Sum/1
  Divide3/1 -> Sum/2
  q/1 -> Divide1/1
  Eg0/1 -> Divide1/2
  k/1 -> Divide1/4
  B/1 -> Divide1/5

== system pv_array2/PV_array /PV module4/PV module/Cel to Kel ==
  "Top " : Inport
  Add : Sum
  Add1 : Sum
  Cel to Kel : Constant  Value=273
  T(ref ^C)1 : Constant  Value=25
  "Tak " : Outport
  "Trk " : Outport  Port=2
  wires:
  Add/1 -> "Tak "/1
  Add1/1 -> "Trk "/1
  T(ref ^C)1/1 -> Add1/1
  Cel to Kel/1 -> Add1/2, Add/2
  "Top "/1 -> Add/1

== system pv_array2/PV_array /PV module4/PV module/NsAkt ==
  TaK : Inport
  Ns : Inport  Port=2
  k : Inport  Port=3
  A : Inport  Port=4
  Product : Product  Inputs=4
  Naskt : Outport
  wires:
  Product/1 -> Naskt/1
  TaK/1 -> Product/4
  Ns/1 -> Product/1
  k/1 -> Product/2
  A/1 -> Product/3

== system pv_array2/PV_array /PV module4/PV module/PV-Panel Current ==
  Is : Inport
  "Vpv " : Inport  Port=2
  NsAkT : Inport  Port=3
  "Iph " : Inport  Port=4
  Np : Inport  Port=5
  q : Inport  Port=6
  Fcn : Fcn  Expr=u(7)*u(2)-u(6)*u(2)*(exp((u(3)*(u(4)+u(5))/u(1)))-1)
  Mux : Mux  Inputs=7
  Rs : Gain  Gain=0.45
  Ipv : Outport
  wires:
  NsAkT/1 -> Mux/1
  Fcn/1 -> Ipv/1, Rs/1
  Rs/1 -> Mux/5
  "Iph "/1 -> Mux/7
  Is/1 -> Mux/6
  "Vpv "/1 -> Mux/4
  Mux/1 -> Fcn/1
  Np/1 -> Mux/2
  q/1 -> Mux/3

== system pv_array2/PV_array /PV module4/PV module/Photon Curr  ==
  "Tak " : Inport
  Trk : Inport  Port=2
  Isc,ref : Inport  Port=3
  "Insolation " : Inport  Port=4
  Ki : Inport  Port=5
  " " : Constant  Value=1000
  Divide : Product  Inputs=*/
  Product : Product
  Product1 : Product
  Sum1 : Sum  Inputs=|++
  Sum2 : Sum  Inputs=|+-
  "Iph " : Outport
  wires:
  "Tak "/1 -> Sum2/1
  Trk/1 -> Sum2/2
  Sum2/1 -> Product/2
  Product/1 -> Sum1/1
  Isc,ref/1 -> Sum1/2
  "Insolation "/1 -> Divide/1
  " "/1 -> Divide/2
  Divide/1 -> Product1/1
  Product1/1 -> "Iph "/1
  Sum1/1 -> Product1/2
  Ki/1 -> Product/1

== system pv_array2/PV_array /PV module4/PV module/Reverse Sat Cur  ==
  "Tak " : Inport
  "Isc ref " : Inport  Port=2
  q : Inport  Port=3
  Voc : Inport  Port=4
  k : Inport  Port=5
  "A " : Inport  Port=6
  "Constant " : Constant
  Divide : Product  Inputs=**////
  Fcn : Fcn  Expr=u(1)/(exp(u(2))-u(3))
  Mux : Mux  Inputs=3
  "Ns " : Constant  Value=36
  Irs : Outport
  wires:
  "Tak "/1 -> Divide/6
  "Ns "/1 -> Divide/4
  "Isc ref "/1 -> Mux/1
  Divide/1 -> Mux/2
  "Constant "/1 -> Mux/3
  Mux/1 -> Fcn/1
  Fcn/1 -> Irs/1
  q/1 -> Divide/1
  Voc/1 -> Divide/2
  k/1 -> Divide/3
  "A "/1 -> Divide/5

== system pv_array2/PV_array /PV module4/PV module/Sat Curr ==
  Irs : Inport
  Tak : Inport  Port=2
  Trk : Inport  Port=3
  q : Inport  Port=4
  Eg0 : Inport  Port=5
  k : Inport  Port=6
  B : Inport  Port=7
  " " : Constant
  Divide : Product  Inputs=*/
  Divide1 : Product  Inputs=***//
  Divide2 : Product  Inputs=*/
  Divide3 : Product  Inputs=*/
  Fcn : Fcn  Expr=(u(1))^3
  Math Function : Math  SaturateOnIntegerOverflow=on
  Product1 : Product  Inputs=3
  Sum : Sum  Inputs=|+-
  Is : Outport
  wires:
  Sum/1 -> Divide1/3
  Fcn/1 -> Product1/2
  Divide/1 -> Fcn/1
  Product1/1 -> Is/1
  Math Function/1 -> Product1/1
  Divide1/1 -> Math Function/1
  Tak/1 -> Divide3/2, Divide/1
  Irs/1 -> Product1/3
  " "/1 -> Divide3/1, Divide2/1
  Trk/1 -> Divide2/2, Divide/2
  Divide2/1 -> Sum/1
  Divide3/1 -> Sum/2
  q/1 -> Divide1/1
  Eg0/1 -> Divide1/2
  k/1 -> Divide1/4
  B/1 -> Divide1/5

== system pv_array2/PV_array /PV module5/PV module/Cel to Kel ==
  "Top " : Inport
  Add : Sum
  Add1 : Sum
  Cel to Kel : Constant  Value=273
  T(ref ^C)1 : Constant  Value=25
  "Tak " : Outport
  "Trk " : Outport  Port=2
  wires:
  Add/1 -> "Tak "/1
  Add1/1 -> "Trk "/1
  T(ref ^C)1/1 -> Add1/1
  Cel to Kel/1 -> Add1/2, Add/2
  "Top "/1 -> Add/1

== system pv_array2/PV_array /PV module5/PV module/NsAkt ==
  TaK : Inport
  Ns : Inport  Port=2
  k : Inport  Port=3
  A : Inport  Port=4
  Product : Product  Inputs=4
  Naskt : Outport
  wires:
  Product/1 -> Naskt/1
  TaK/1 -> Product/4
  Ns/1 -> Product/1
  k/1 -> Product/2
  A/1 -> Product/3

== system pv_array2/PV_array /PV module5/PV module/PV-Panel Current ==
  Is : Inport
  "Vpv " : Inport  Port=2
  NsAkT : Inport  Port=3
  "Iph " : Inport  Port=4
  Np : Inport  Port=5
  q : Inport  Port=6
  Fcn : Fcn  Expr=u(7)*u(2)-u(6)*u(2)*(exp((u(3)*(u(4)+u(5))/u(1)))-1)
  Mux : Mux  Inputs=7
  Rs : Gain  Gain=0.45
  Ipv : Outport
  wires:
  NsAkT/1 -> Mux/1
  Fcn/1 -> Ipv/1, Rs/1
  Rs/1 -> Mux/5
  "Iph "/1 -> Mux/7
  Is/1 -> Mux/6
  "Vpv "/1 -> Mux/4
  Mux/1 -> Fcn/1
  Np/1 -> Mux/2
  q/1 -> Mux/3

== system pv_array2/PV_array /PV module5/PV module/Photon Curr  ==
  "Tak " : Inport
  Trk : Inport  Port=2
  Isc,ref : Inport  Port=3
  "Insolation " : Inport  Port=4
  Ki : Inport  Port=5
  " " : Constant  Value=1000
  Divide : Product  Inputs=*/
  Product : Product
  Product1 : Product
  Sum1 : Sum  Inputs=|++
  Sum2 : Sum  Inputs=|+-
  "Iph " : Outport
  wires:
  "Tak "/1 -> Sum2/1
  Trk/1 -> Sum2/2
  Sum2/1 -> Product/2
  Product/1 -> Sum1/1
  Isc,ref/1 -> Sum1/2
  "Insolation "/1 -> Divide/1
  " "/1 -> Divide/2
  Divide/1 -> Product1/1
  Product1/1 -> "Iph "/1
  Sum1/1 -> Product1/2
  Ki/1 -> Product/1

== system pv_array2/PV_array /PV module5/PV module/Reverse Sat Cur  ==
  "Tak " : Inport
  "Isc ref " : Inport  Port=2
  q : Inport  Port=3
  Voc : Inport  Port=4
  k : Inport  Port=5
  "A " : Inport  Port=6
  "Constant " : Constant
  Divide : Product  Inputs=**////
  Fcn : Fcn  Expr=u(1)/(exp(u(2))-u(3))
  Mux : Mux  Inputs=3
  "Ns " : Constant  Value=36
  Irs : Outport
  wires:
  "Tak "/1 -> Divide/6
  "Ns "/1 -> Divide/4
  "Isc ref "/1 -> Mux/1
  Divide/1 -> Mux/2
  "Constant "/1 -> Mux/3
  Mux/1 -> Fcn/1
  Fcn/1 -> Irs/1
  q/1 -> Divide/1
  Voc/1 -> Divide/2
  k/1 -> Divide/3
  "A "/1 -> Divide/5

== system pv_array2/PV_array /PV module5/PV module/Sat Curr ==
  Irs : Inport
  Tak : Inport  Port=2
  Trk : Inport  Port=3
  q : Inport  Port=4
  Eg0 : Inport  Port=5
  k : Inport  Port=6
  B : Inport  Port=7
  " " : Constant
  Divide : Product  Inputs=*/
  Divide1 : Product  Inputs=***//
  Divide2 : Product  Inputs=*/
  Divide3 : Product  Inputs=*/
  Fcn : Fcn  Expr=(u(1))^3
  Math Function : Math  SaturateOnIntegerOverflow=on
  Product1 : Product  Inputs=3
  Sum : Sum  Inputs=|+-
  Is : Outport
  wires:
  Sum/1 -> Divide1/3
  Fcn/1 -> Product1/2
  Divide/1 -> Fcn/1
  Product1/1 -> Is/1
  Math Function/1 -> Product1/1
  Divide1/1 -> Math Function/1
  Tak/1 -> Divide3/2, Divide/1
  Irs/1 -> Product1/3
  " "/1 -> Divide3/1, Divide2/1
  Trk/1 -> Divide2/2, Divide/2
  Divide2/1 -> Sum/1
  Divide3/1 -> Sum/2
  q/1 -> Divide1/1
  Eg0/1 -> Divide1/2
  k/1 -> Divide1/4
  B/1 -> Divide1/5

== system pv_array2/PV_array /PV module6/PV module/Cel to Kel ==
  "Top " : Inport
  Add : Sum
  Add1 : Sum
  Cel to Kel : Constant  Value=273
  T(ref ^C)1 : Constant  Value=25
  "Tak " : Outport
  "Trk " : Outport  Port=2
  wires:
  Add/1 -> "Tak "/1
  Add1/1 -> "Trk "/1
  T(ref ^C)1/1 -> Add1/1
  Cel to Kel/1 -> Add1/2, Add/2
  "Top "/1 -> Add/1

== system pv_array2/PV_array /PV module6/PV module/NsAkt ==
  TaK : Inport
  Ns : Inport  Port=2
  k : Inport  Port=3
  A : Inport  Port=4
  Product : Product  Inputs=4
  Naskt : Outport
  wires:
  Product/1 -> Naskt/1
  TaK/1 -> Product/4
  Ns/1 -> Product/1
  k/1 -> Product/2
  A/1 -> Product/3

== system pv_array2/PV_array /PV module6/PV module/PV-Panel Current ==
  Is : Inport
  "Vpv " : Inport  Port=2
  NsAkT : Inport  Port=3
  "Iph " : Inport  Port=4
  Np : Inport  Port=5
  q : Inport  Port=6
  Fcn : Fcn  Expr=u(7)*u(2)-u(6)*u(2)*(exp((u(3)*(u(4)+u(5))/u(1)))-1)
  Mux : Mux  Inputs=7
  Rs : Gain  Gain=0.45
  Ipv : Outport
  wires:
  NsAkT/1 -> Mux/1
  Fcn/1 -> Ipv/1, Rs/1
  Rs/1 -> Mux/5
  "Iph "/1 -> Mux/7
  Is/1 -> Mux/6
  "Vpv "/1 -> Mux/4
  Mux/1 -> Fcn/1
  Np/1 -> Mux/2
  q/1 -> Mux/3
